simulink model "untitled"  (R2021b)
settings: Solver=VariableStepAuto  StartTime=0.0  StopTime=30  MaxStep=0.1  RelTol=1e-3
values from neighbouring files (symbols this model uses):
  d = 4.7    [parameter.m]
  p = m*l^2+J    (= 2.452)    [parameter.m]
  r = m*g*l    (= 16.8)    [parameter.m]
settings Model: Creator=the_main_notebook  LastModifiedBy=the_main_notebook
settings SolverCC: InitialStep=0.01

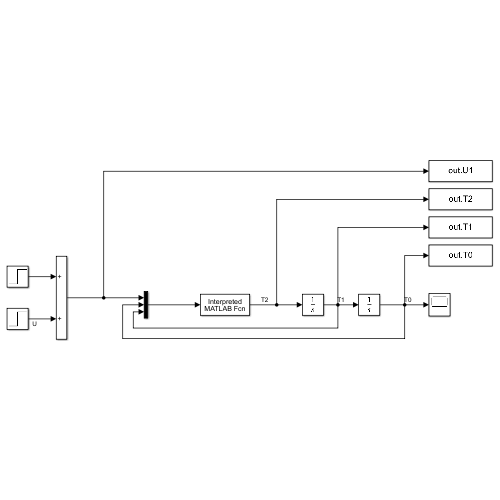
[thumbnail: Simulink's stored preview of the top-level diagram]
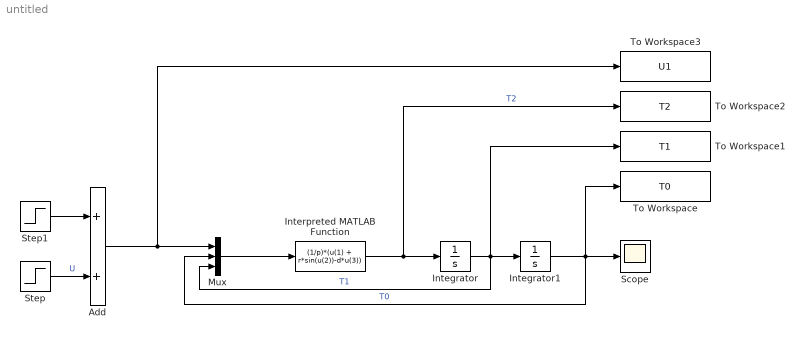
== system untitled ==
  Add : Sum
  Integrator : Integrator
  Integrator1 : Integrator
  Interpreted MATLAB Function : MATLABFcn  MATLABFcn=(1/p)*(u(1) + r*sin(u(2))-d*u(3))
  Mux : Mux  Inputs=3
  Scope : Scope
  Step : Step  SampleTime=0
  Step1 : Step  Time=15  After=5  SampleTime=0
  To Workspace : ToWorkspace  VariableName=T0  SaveFormat=Timeseries  SampleTime=-1
  To Workspace1 : ToWorkspace  VariableName=T1  SaveFormat=Timeseries  SampleTime=-1
  To Workspace2 : ToWorkspace  VariableName=T2  SaveFormat=Timeseries  SampleTime=-1
  To Workspace3 : ToWorkspace  VariableName=U1  SaveFormat=Timeseries  SampleTime=-1
  wires:
  Interpreted MATLAB Function/1 -> To Workspace2/1, Integrator/1  "T2"
  Integrator/1 -> Integrator1/1, To Workspace1/1, Mux/3  "T1"
  Mux/1 -> Interpreted MATLAB Function/1
  Integrator1/1 -> To Workspace/1, Scope/1, Mux/2  "T0"
  Step/1 -> Add/2  "U"
  Add/1 -> To Workspace3/1, Mux/1
  Step1/1 -> Add/1
